simulink model "dpt_vektor_matr"  (R2021b)
settings: Solver=VariableStepAuto  StartTime=0.0  StopTime=0.4  RelTol=1e-3
values from neighbouring files (symbols this model uses):
  Jn = 2*Jd    (= 3.92e-05)    [pasport_dpt.m]
  ke = (Un-R*In)/wn    (= 0.236312997347)    [pasport_dpt.m]
  km = Mn/In    (= 0.156097560976)    [pasport_dpt.m]
  ku = 20    [pasport_dpt.m]
  L = 10^-3*140    (= 0.14)    [pasport_dpt.m]
  R = 51    [pasport_dpt.m]
settings Model: Creator=Admin  LastModifiedBy=Admin

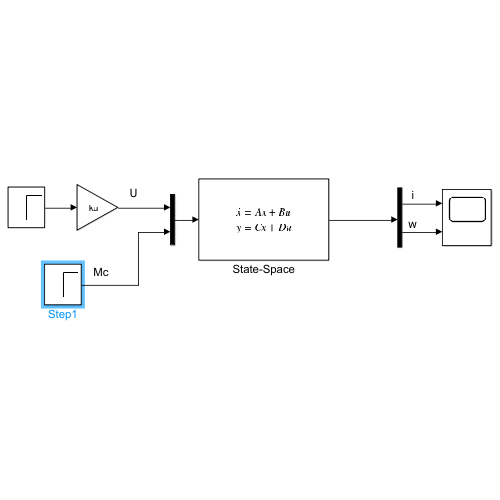
[thumbnail: Simulink's stored preview of the top-level diagram]
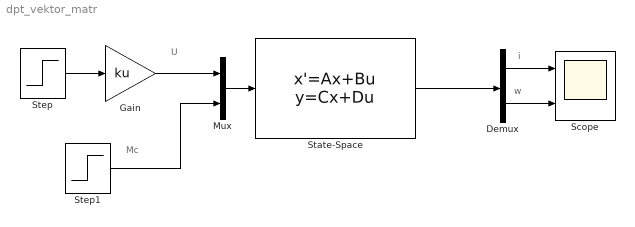
== system dpt_vektor_matr ==
  note: Mc
  note: i
  note: w
  note: U
  Demux : Demux  Outputs=2
  Gain : Gain  Gain=ku
  Mux : Mux  Inputs=2
  Scope : Scope  NumInputPorts=2
  State-Space : StateSpace  A=[-R/L -ke/L; km/Jn 0]  B=[1/L 0; 0 -1/Jn]  C=[km 0; 0 1]  D=zeros(2,2)  InitialCondition=0
  Step : Step  Time=0  SampleTime=0
  Step1 : Step  Time=0.35  After=0.02  SampleTime=0  VectorParams1D=off  ZeroCross=off
  wires:
  State-Space/1 -> Demux/1
  Step/1 -> Gain/1
  Mux/1 -> State-Space/1
  Demux/1 -> Scope/1
  Demux/2 -> Scope/2
  Gain/1 -> Mux/1
  Step1/1 -> Mux/2
